simulink model "MPC_CelltesterV1"  (R2019a)
settings: Solver=VariableStepAuto  StartTime=0.0  StopTime=5000  RelTol=2e-14
undefined symbols (not defined in the file or in its folder): Ion, Lithium
libraries: powerlib x31, simulink x2, electricdrivelib x1
settings Model: Creator=kagom  LastModifiedBy=kagom
settings SolverCC: ZeroCrossAlgorithm=Adaptive
settings OptimizationCC: EfficientMapNaN2IntZero=off
settings DebuggingCC: IgnoredZcDiagnostic=none
settings HardwareCC: TargetBitPerPointer=64  TargetBitPerSizeT=64  TargetBitPerPtrDiffT=64  TargetLongLongMode=on  TargetIntDivRoundTo=Zero  TargetEndianess=LittleEndian  TargetWordSize=64  TargetHWDeviceType=MATLAB Host  ProdEqTarget=off
settings CodeAppCC: MaxIdLength=128
settings GRTTargetCC: TargetLangStandard=C89/C90 (ANSI)  GRTInterface=on

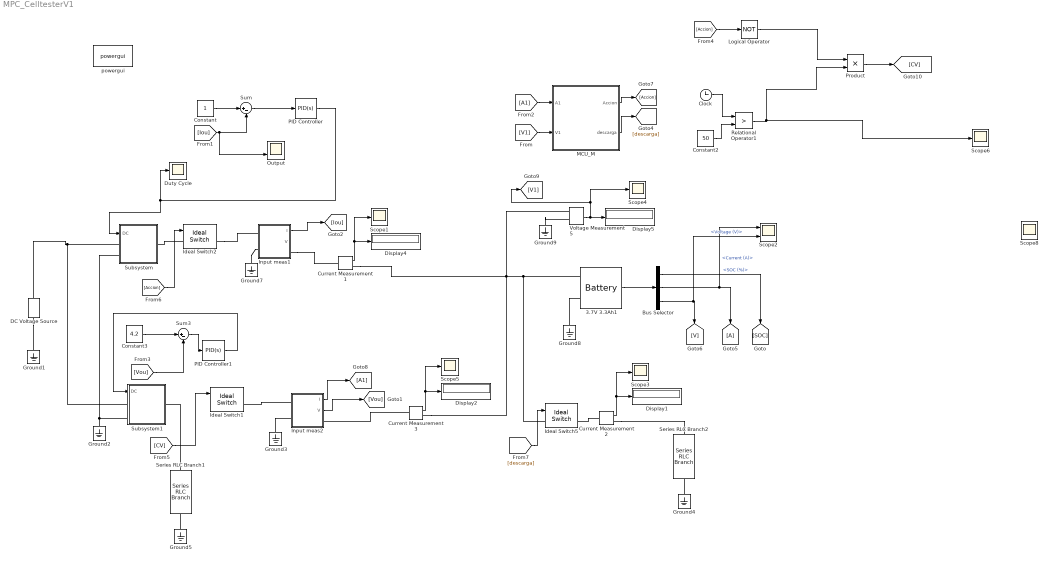
== system MPC_CelltesterV1 ==
  3.7V 3.3Ah1 : electricdrivelib/Extra Sources/Battery  BatType=Lithium-Ion  ShowTempParam=off  ThermalPreset=no  ShowAgeParam=off  NomV=3.7  NomQ=3.3  SOC=98  Batt_Tr=1  PresetModel=off  MaxQ=3.3  MinV=2.5  FullV=4.2  Dis_rate=1.0  R=0.010909  Normal_OP=2.9843  expZone="[3.8894     0.16213]"  current=[6.5 13 32.5]  Units=Ampere-hour  Tci=20  NomT=20  T2=-30  MaxQ2=4.8  FullV2=7.1  Normal_OP2=5.655  expZone2="[6.58           1]"  Rca=0.6  ti=2000  Dp=0  Neq0=0  Tsim=1e6  Ta1=25  Qeol=5.4*0.9  Reol=0.013333*1.2  Char_age=[2.3478, 3]  Dis_age=[2.3478, 10]  N1=1500  N2=10500  N3=1000  N4=1400  Ta2=45  N5=950
      settings: SourceProductName=Simscape Electrical
  Bus Selector : BusSelector  OutputSignals=SOC (%),Current (A),Voltage (V)
  Clock : Clock
  Constant : Constant
  Constant2 : Constant  Value=50
  Constant3 : Constant  Value=4.2
  Current Measurement1 : powerlib/Measurements/Current Measurement  PhasorSimulation=off  OutputType=Complex  PSBequivalent=0
      settings: SourceProductName=Simscape Electrical
  Current Measurement2 : powerlib/Measurements/Current Measurement  PhasorSimulation=off  OutputType=Complex  PSBequivalent=0
      settings: SourceProductName=Simscape Electrical
  Current Measurement3 : powerlib/Measurements/Current Measurement  PhasorSimulation=off  OutputType=Complex  PSBequivalent=0
      settings: SourceProductName=Simscape Electrical
  DC Voltage Source : powerlib/Electrical Sources/DC Voltage Source  Amplitude=5  Measurements=None
      settings: SourceProductName=Simscape Electrical
  Display{1..2,4..5} (4 alike) : Display
  Duty Cycle : Scope
  Ground{1..5,7..9} (8 alike) : powerlib/Elements/Ground  LConnTagsString=a
      settings: SourceProductName=Simscape Electrical
  Ideal Switch1 : powerlib/Power Electronics/Ideal Switch  Ron=0.001  Lon=0  IC=0  Rs=1e5  Cs=inf  Measurements=on
      settings: SourceProductName=Simscape Electrical
  Ideal Switch2 : powerlib/Power Electronics/Ideal Switch  Ron=0.001  Lon=0  IC=1  Rs=1e5  Cs=inf  Measurements=on
      settings: SourceProductName=Simscape Electrical
  Ideal Switch5 : powerlib/Power Electronics/Ideal Switch  Ron=0.001  Lon=0  IC=0  Rs=1e5  Cs=inf  Measurements=on
      settings: SourceProductName=Simscape Electrical
  Input meas1 : Subsystem
  Input meas2 : Subsystem
  Logical Operator : Logic  Operator=NOT  AllPortsSameDT=off  OutDataTypeStr=boolean
  MCU_M : Stateflow chart  TreatAsAtomicUnit=on
  Output : Scope  NumInputPorts=2
  PID Controller : simulink/Continuous/PID Controller  Controller=PID  Form=Parallel  TimeDomain=Continuous-time  SampleTime=-1  IntegratorMethod=Forward Euler  FilterMethod=Forward Euler  ControllerParametersSource=internal  P=1  I=1  D=0  UseFilter=on  N=100  TunerSelectOption=Frequency Response Based  InitialConditionSource=internal  InitialConditionForIntegrator=0  InitialConditionForFilter=0  DifferentiatorICPrevScaledInput=0  ExternalReset=none  TrackingMode=off  Kt=1  LimitOutput=on  UpperSaturationLimit=0.9  LowerSaturationLimit=0.1  LinearizeAsGain=on  AntiWindupMode=none  Kb=1  POutMin=[]  POutMax=[]  IOutMin=[]  IOutMax=[]  DOutMin=[]  DOutMax=[]  NOutMin=[]  NOutMax=[]  SumOutMin=[]  SumOutMax=[]  SaturationOutMin=[]  SaturationOutMax=[]  PParamMin=[]  PParamMax=[]  IParamMin=[]  IParamMax=[]  DParamMin=[]  DParamMax=[]  NParamMin=[]  NParamMax=[]  KbParamMin=[]  KbParamMax=[]  KtParamMin=[]  KtParamMax=[]  KbOutMin=[]  KbOutMax=[]  KtOutMin=[]  KtOutMax=[]  IntegratorOutMin=[]  IntegratorOutMax=[]  FilterOutMin=[]  FilterOutMax=[]  SumI1OutMin=[]  SumI1OutMax=[]  SumI2OutMin=[]  SumI2OutMax=[]  SumI3OutMin=[]  SumI3OutMax=[]  SumI4OutMin=[]  SumI4OutMax=[]  SumDOutMin=[]  SumDOutMax=[]  DifferentiatorOutMin=[]  DifferentiatorOutMax=[]  FilterDiffOutCoefMin=[]  FilterDiffOutCoefMax=[]  ReciprocalOutMin=[]  ReciprocalOutMax=[]  SumDenOutMin=[]  SumDenOutMax=[]  SumNumOutMin=[]  SumNumOutMax=[]  DivideOutMin=[]  DivideOutMax=[]  IntegratorContinuousStateAttributes=''  IntegratorStateMustResolveToSignalObject=off  IntegratorRTWStateStorageClass=Auto  FilterContinuousStateAttributes=''  FilterStateMustResolveToSignalObject=off  FilterRTWStateStorageClass=Auto  ParallelPVariant=InternalParameters  IdealPVariant=Disabled  IVariant=InternalParameters  DVariant=InternalParameters  IntegratorVariant=Continuous  SatVariant=Enabled  AWVariant=Passthrough  PCopyVariant=Disabled  TRVariant=Disabled  FdbkBlocksVariant=Forward  IdealPFdbkVariant=Disabled  SatFdbkVariant=Disabled  DerivativeFilterVariant=ContFilter  NVariant=InternalParameters  NCopyVariant=Disabled  FilterICVariant=InternalICsFilter  IntegratorICVariant=InternalICs  ExternalResetVariant=Disabled  TRSumVariant=Passthrough  SumFdbkVariant=Disabled  SumVariant=Sum_PID
  PID Controller1 : simulink/Continuous/PID Controller  Controller=PID  Form=Parallel  TimeDomain=Continuous-time  SampleTime=-1  IntegratorMethod=Forward Euler  FilterMethod=Forward Euler  ControllerParametersSource=internal  P=1  I=1  D=0  UseFilter=on  N=100  TunerSelectOption=Frequency Response Based  InitialConditionSource=internal  InitialConditionForIntegrator=0  InitialConditionForFilter=0  DifferentiatorICPrevScaledInput=0  ExternalReset=none  TrackingMode=off  Kt=1  LimitOutput=on  UpperSaturationLimit=0.9  LowerSaturationLimit=0.1  LinearizeAsGain=on  AntiWindupMode=none  Kb=1  POutMin=[]  POutMax=[]  IOutMin=[]  IOutMax=[]  DOutMin=[]  DOutMax=[]  NOutMin=[]  NOutMax=[]  SumOutMin=[]  SumOutMax=[]  SaturationOutMin=[]  SaturationOutMax=[]  PParamMin=[]  PParamMax=[]  IParamMin=[]  IParamMax=[]  DParamMin=[]  DParamMax=[]  NParamMin=[]  NParamMax=[]  KbParamMin=[]  KbParamMax=[]  KtParamMin=[]  KtParamMax=[]  KbOutMin=[]  KbOutMax=[]  KtOutMin=[]  KtOutMax=[]  IntegratorOutMin=[]  IntegratorOutMax=[]  FilterOutMin=[]  FilterOutMax=[]  SumI1OutMin=[]  SumI1OutMax=[]  SumI2OutMin=[]  SumI2OutMax=[]  SumI3OutMin=[]  SumI3OutMax=[]  SumI4OutMin=[]  SumI4OutMax=[]  SumDOutMin=[]  SumDOutMax=[]  DifferentiatorOutMin=[]  DifferentiatorOutMax=[]  FilterDiffOutCoefMin=[]  FilterDiffOutCoefMax=[]  ReciprocalOutMin=[]  ReciprocalOutMax=[]  SumDenOutMin=[]  SumDenOutMax=[]  SumNumOutMin=[]  SumNumOutMax=[]  DivideOutMin=[]  DivideOutMax=[]  IntegratorContinuousStateAttributes=''  IntegratorStateMustResolveToSignalObject=off  IntegratorRTWStateStorageClass=Auto  FilterContinuousStateAttributes=''  FilterStateMustResolveToSignalObject=off  FilterRTWStateStorageClass=Auto  ParallelPVariant=InternalParameters  IdealPVariant=Disabled  IVariant=InternalParameters  DVariant=InternalParameters  IntegratorVariant=Continuous  SatVariant=Enabled  AWVariant=Passthrough  PCopyVariant=Disabled  TRVariant=Disabled  FdbkBlocksVariant=Forward  IdealPFdbkVariant=Disabled  SatFdbkVariant=Disabled  DerivativeFilterVariant=ContFilter  NVariant=InternalParameters  NCopyVariant=Disabled  FilterICVariant=InternalICsFilter  IntegratorICVariant=InternalICs  ExternalResetVariant=Disabled  TRSumVariant=Passthrough  SumFdbkVariant=Disabled  SumVariant=Sum_PID
  Product : Product
  Relational Operator1 : RelationalOperator  Operator=>  OutDataTypeStr=boolean  RndMeth=Simplest
  Scope{1,3..6,8} (6 alike) : Scope
  Scope2 : Scope  NumInputPorts=2
  Series RLC Branch1 : powerlib/Elements/Series RLC Branch  LConnTagsString=__new0  RConnTagsString=__new0  BranchType=R  Resistance=100000  Inductance=1e-3  SetiL0=off  InitialCurrent=0  Capacitance=1e-6  Setx0=off  InitialVoltage=0  Measurements=None
      settings: SourceProductName=Simscape Electrical
  Series RLC Branch2 : powerlib/Elements/Series RLC Branch  LConnTagsString=__new0  RConnTagsString=__new0  BranchType=R  Resistance=10  Inductance=1e-3  SetiL0=off  InitialCurrent=0  Capacitance=1e-6  Setx0=off  InitialVoltage=0  Measurements=None
      settings: SourceProductName=Simscape Electrical
  Subsystem : Subsystem
  Subsystem1 : Subsystem
  Sum : Sum  Inputs=|+-
  Sum3 : Sum  Inputs=|+-
  Voltage Measurement5 : powerlib/Measurements/Voltage Measurement  PhasorSimulation=off  OutputType=Complex  PSBequivalent=0
      settings: SourceProductName=Simscape Electrical
  powergui : powerlib/powergui  Priority=1  SimulationMode=Continuous  SampleTime=1e-3  frequency=60  Iterations=50  frequencyindice=0  Pbase=100e6  ErrMax=1e-4  UnitsV=kV  UnitsW=MW  buscounter=0  FunctionMessages=off  echomessages=off  EnableUseOfTLC=off  CurrentSourceSwitches=off  DisableSnubberDevices=off  DisableRonSwitches=off  DisableVfSwitches=off  DisplayEquations=off  AutomaticDiscreteSolvers=off  SolverType=Tustin/Backward Euler (TBE)  Interpol=off  ExternalGateDelay=off  methode=off  Ts=100  x0status=blocks  SPID=on  SwTol=0  HookPort=off  NonlinearTolerance=0  nMaxIteration=15  ContinueOnMaxIteration=off  RestoreLinks=warning  ResistiveCurrentMeasurement=off  Frange=[0:2:500]  Ylog=off  Xlog=on  ShowGrid=off  save=off  variable=ZData  structure=0  ZoomFFT=off  StartTime=0.0  cycles=1  DisplayStyle=1  fundamental=60  FreqAxis=off  MaxFrequency=1000  frequencyindicesteady=1  RmsSteady=1  display=off
      settings: SourceProductName=Simscape Electrical
  wires:
  Constant3/1 -> Sum3/1
  Sum3/1 -> PID Controller1/1
  [Iou] -> Output/2, Sum/2
  Constant/1 -> Sum/1
  Sum/1 -> PID Controller/1
  Input meas1/1(I) -> [Iou]
  Current Measurement1/1 -> Scope1/1, Display4/1
  PID Controller/1 -> Duty Cycle/1, Subsystem/1(DC)
  PID Controller1/1 -> Subsystem1/1(DC)
  3.7V 3.3Ah1/1 -> Bus Selector/1
  Bus Selector/1 -> [SOC]  "<SOC (%)>"
  Bus Selector/3 -> Scope2/2, [V]  "<Voltage (V)>"
  Bus Selector/2 -> Scope2/1, [A]  "<Current (A)>"
  [V1] -> MCU_M/2(V1)
  MCU_M/1(Accion) -> [Accion]
  [Vou] -> Sum3/2
  Input meas2/2(V) -> [Vou]
  [A1] -> MCU_M/1(A1)
  [Accion] -> Ideal Switch2/1
  [CV] -> Ideal Switch1/1
  MCU_M/2(descarga) -> [descarga]
  [descarga] -> Ideal Switch5/1
  Current Measurement2/1 -> Scope3/1, Display1/1
  Current Measurement3/1 -> Scope5/1, Display2/1
  Input meas2/1(I) -> [A1]
  Voltage Measurement5/1 -> Scope4/1, [V1], Display5/1
  Clock/1 -> Relational Operator1/1
  [Accion] -> Logical Operator/1
  Relational Operator1/1 -> Product/2, Scope6/1
  Constant2/1 -> Relational Operator1/2
  Logical Operator/1 -> Product/1
  Product/1 -> [CV]
  connections:
  Ground7/LConn1 -- Input meas1/LConn2
  Ground9/LConn1 -- Voltage Measurement5/LConn2
  Ground8/LConn1 -- 3.7V 3.3Ah1/LConn2
  Input meas1/RConn1 -- Current Measurement1/LConn1
  DC Voltage Source/LConn1 -- Ground1/LConn1
  DC Voltage Source/RConn1 -- Subsystem1/LConn1 -- Subsystem/LConn1
  Ground2/LConn1 -- Subsystem1/LConn2 -- Subsystem/LConn2
  Ground3/LConn1 -- Input meas2/LConn2
  Series RLC Branch1/LConn1 -- Subsystem1/RConn1
  Ideal Switch2/LConn1 -- Subsystem/RConn1
  Ideal Switch2/RConn1 -- Input meas1/LConn1
  Input meas2/LConn1 -- Ideal Switch1/RConn1
  Ground4/LConn1 -- Series RLC Branch2/RConn1
  Voltage Measurement5/LConn1 -- Current Measurement3/RConn1 -- Current Measurement1/RConn1 -- Ideal Switch5/LConn1 -- 3.7V 3.3Ah1/LConn1
  Current Measurement2/LConn1 -- Ideal Switch5/RConn1
  Current Measurement2/RConn1 -- Series RLC Branch2/LConn1
  Current Measurement3/LConn1 -- Input meas2/RConn1
  Ground5/LConn1 -- Series RLC Branch1/RConn1

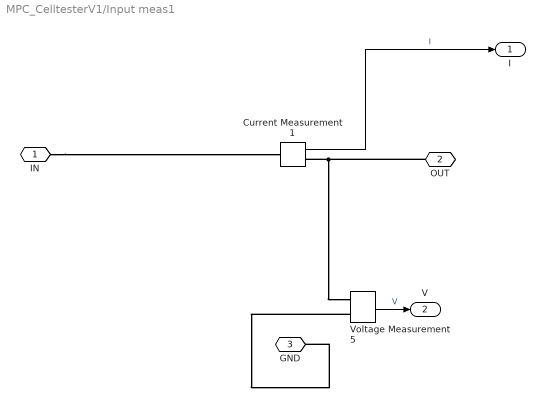
== system MPC_CelltesterV1/Input meas1 ==
  Current Measurement1 : powerlib/Measurements/Current Measurement  PhasorSimulation=off  OutputType=Complex  PSBequivalent=0
      settings: SourceProductName=Simscape Electrical
  Voltage Measurement5 : powerlib/Measurements/Voltage Measurement  PhasorSimulation=off  OutputType=Complex  PSBequivalent=0
      settings: SourceProductName=Simscape Electrical
  IN : PMIOPort  Side=Left
  OUT : PMIOPort  Port=2  Side=Right
  GND : PMIOPort  Port=3  Side=Left
  I : Outport  VectorParamsAs1DForOutWhenUnconnected=on
  V : Outport  Port=2  VectorParamsAs1DForOutWhenUnconnected=on
  wires:
  Current Measurement1/1 -> I/1  "I"
  Voltage Measurement5/1 -> V/1  "V"
  connections:
  OUT/RConn1 -- Current Measurement1/RConn1 -- Voltage Measurement5/LConn1
  Voltage Measurement5/LConn2 -- GND/RConn1
  IN/RConn1 -- Current Measurement1/LConn1

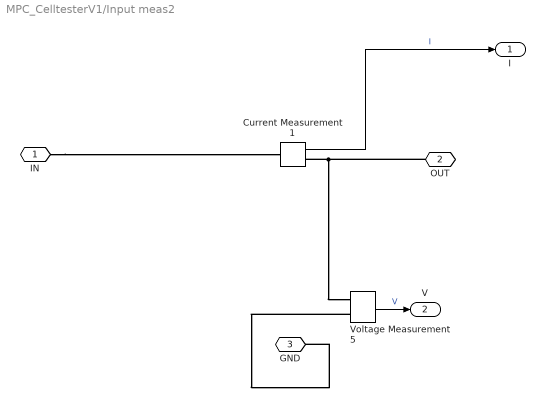
== system MPC_CelltesterV1/Input meas2 ==
  Current Measurement1 : powerlib/Measurements/Current Measurement  PhasorSimulation=off  OutputType=Complex  PSBequivalent=0
      settings: SourceProductName=Simscape Electrical
  Voltage Measurement5 : powerlib/Measurements/Voltage Measurement  PhasorSimulation=off  OutputType=Complex  PSBequivalent=0
      settings: SourceProductName=Simscape Electrical
  IN : PMIOPort  Side=Left
  OUT : PMIOPort  Port=2  Side=Right
  GND : PMIOPort  Port=3  Side=Left
  I : Outport  VectorParamsAs1DForOutWhenUnconnected=on
  V : Outport  Port=2  VectorParamsAs1DForOutWhenUnconnected=on
  wires:
  Current Measurement1/1 -> I/1  "I"
  Voltage Measurement5/1 -> V/1  "V"
  connections:
  OUT/RConn1 -- Current Measurement1/RConn1 -- Voltage Measurement5/LConn1
  Voltage Measurement5/LConn2 -- GND/RConn1
  IN/RConn1 -- Current Measurement1/LConn1

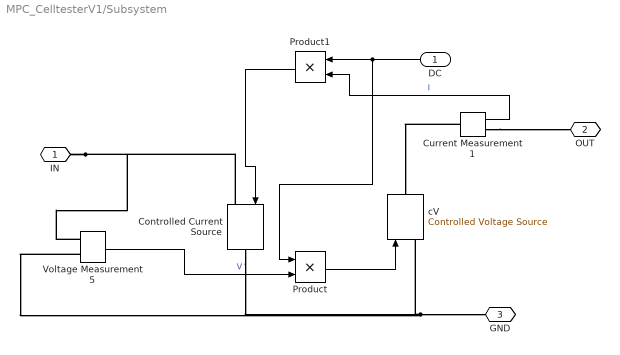
== system MPC_CelltesterV1/Subsystem ==
  DC : Inport
  Controlled Current Source : powerlib/Electrical Sources/Controlled Current Source  Initialize=on  Source_Type=DC  Amplitude=0  Phase=0  Frequency=0  Measurements=None
      settings: SourceProductName=Simscape Electrical
  Current Measurement1 : powerlib/Measurements/Current Measurement  PhasorSimulation=off  OutputType=Complex  PSBequivalent=0
      settings: SourceProductName=Simscape Electrical
  Product : Product
  Product1 : Product
  Voltage Measurement5 : powerlib/Measurements/Voltage Measurement  PhasorSimulation=off  OutputType=Complex  PSBequivalent=0
      settings: SourceProductName=Simscape Electrical
  cV : powerlib/Electrical Sources/Controlled Voltage Source  Initialize=on  Source_Type=DC  Amplitude=0  Phase=0  Frequency=0  Measurements=None
      settings: SourceProductName=Simscape Electrical
  IN : PMIOPort  Side=Left
  OUT : PMIOPort  Port=2  Side=Right
  GND : PMIOPort  Port=3  Side=Left
  wires:
  Voltage Measurement5/1 -> Product/2  "V"
  DC/1 -> Product/1, Product1/1
  Current Measurement1/1 -> Product1/2  "I"
  Product/1 -> cV/1
  Product1/1 -> Controlled Current Source/1
  connections:
  Current Measurement1/LConn1 -- cV/RConn1
  IN/RConn1 -- Controlled Current Source/LConn1 -- Voltage Measurement5/LConn1
  Current Measurement1/RConn1 -- OUT/RConn1
  Controlled Current Source/RConn1 -- Voltage Measurement5/LConn2 -- cV/LConn1 -- GND/RConn1

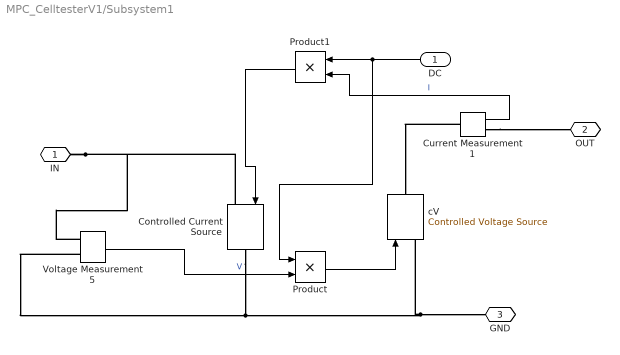
== system MPC_CelltesterV1/Subsystem1 ==
  DC : Inport
  Controlled Current Source : powerlib/Electrical Sources/Controlled Current Source  Initialize=on  Source_Type=DC  Amplitude=0  Phase=0  Frequency=0  Measurements=None
      settings: SourceProductName=Simscape Electrical
  Current Measurement1 : powerlib/Measurements/Current Measurement  PhasorSimulation=off  OutputType=Complex  PSBequivalent=0
      settings: SourceProductName=Simscape Electrical
  Product : Product
  Product1 : Product
  Voltage Measurement5 : powerlib/Measurements/Voltage Measurement  PhasorSimulation=off  OutputType=Complex  PSBequivalent=0
      settings: SourceProductName=Simscape Electrical
  cV : powerlib/Electrical Sources/Controlled Voltage Source  Initialize=on  Source_Type=DC  Amplitude=0  Phase=0  Frequency=0  Measurements=None
      settings: SourceProductName=Simscape Electrical
  IN : PMIOPort  Side=Left
  OUT : PMIOPort  Port=2  Side=Right
  GND : PMIOPort  Port=3  Side=Left
  wires:
  Voltage Measurement5/1 -> Product/2  "V"
  DC/1 -> Product/1, Product1/1
  Current Measurement1/1 -> Product1/2  "I"
  Product/1 -> cV/1
  Product1/1 -> Controlled Current Source/1
  connections:
  Current Measurement1/LConn1 -- cV/RConn1
  IN/RConn1 -- Controlled Current Source/LConn1 -- Voltage Measurement5/LConn1
  Current Measurement1/RConn1 -- OUT/RConn1
  Controlled Current Source/RConn1 -- Voltage Measurement5/LConn2 -- cV/LConn1 -- GND/RConn1

== stateflow chart MPC_CelltesterV1/MCU_M ==
  state CC
    entry : Accion = 1
  state CV
    entry : Accion = 0
  state Carga
    entry : descarga = 1
  state Descarga
    entry : descarga  = 0
  (default) -> CC [order 1]
  CC -> CV : [V1>4.2]
  CV -> CC : [V1<2.5]
  (default) -> Carga [order 2]
  Carga -> Descarga : [A1<0.1]
  Descarga -> Carga : [V1<2.5]
  data: Accion output; A1 input; descarga output; V1 input
